simulink model "ClosedLoop_Cq"  (R2023b)
settings: Solver=VariableStepAuto  StartTime=0.0  StopTime=10.0  RelTol=1e-3
libraries: cstblocks x3
settings Model: Creator=PierluigiMeneses  LastModifiedBy=Antonio

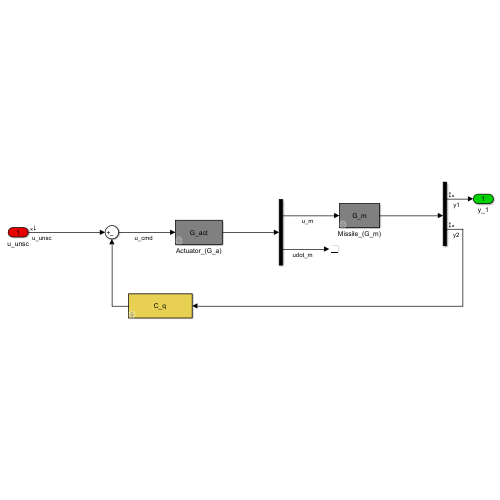
[thumbnail: Simulink's stored preview of the top-level diagram]
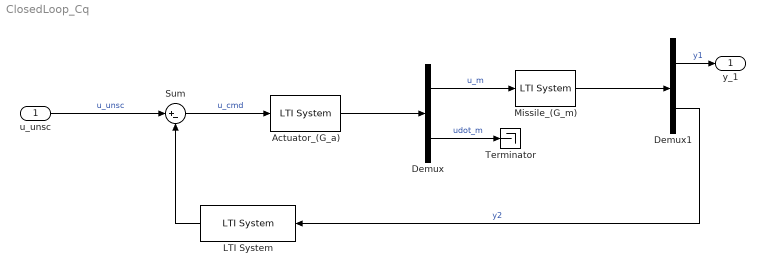
== system ClosedLoop_Cq ==
  u_unsc : Inport
  Actuator_(G_a) : cstblocks/LTI System  sys=G_act  IC=[]  PadeOrder=0
  Demux : Demux  Outputs=2
  Demux1 : Demux  Outputs=2
  LTI System : cstblocks/LTI System  sys=C_q  IC=[]  PadeOrder=0
  Missile_(G_m) : cstblocks/LTI System  sys=G_m  IC=[]  PadeOrder=0
  Sum : Sum  Inputs=|+-
  Terminator : Terminator
  y_1 : Outport
  wires:
  Demux1/1 -> y_1/1  "y1"
  Demux/1 -> Missile_(G_m)/1  "u_m"
  Demux1/2 -> LTI System/1  "y2"
  Demux/2 -> Terminator/1  "udot_m"
  Missile_(G_m)/1 -> Demux1/1
  Actuator_(G_a)/1 -> Demux/1
  LTI System/1 -> Sum/2
  u_unsc/1 -> Sum/1  "u_unsc"
  Sum/1 -> Actuator_(G_a)/1  "u_cmd"
